simulink library "fuzblock"  (Simulink 6.0)
settings: Solver=ode45  SolverMode=SingleTasking  StartTime=0.0  StopTime=10.0  RelTol=1e-3
values from neighbouring files (symbols this model uses):
  fis = setfis(fis,'ruleList',newRuleList)    [addrule.m]    (also in anfsedit.m = get(gcbf,'UserData'); cmfdlg.m = addmf(fis,varType,varIndex,mfName,mfType,mfParams); cmthdlg.m = setfield(fis,methodType,methodName); fisgui.m = oldfis{1})
libraries: fuzblock x6
settings Model: CovMetricSettings=d  Creator=sanjai  LastModifiedBy=pascal  ProdHWDeviceType=Specified
settings DataIOCC: SignalLoggingName=logsOut
settings OptimizationCC: BooleanDataType=off
settings DebuggingCC: CheckExecutionContextPreStartOutputMsg=on  CheckExecutionContextRuntimeOutputMsg=on  SolverPrmCheckMsg=none
settings HardwareCC: ProdHWDeviceType=Specified
settings GRTTargetCC: UtilityFuncGeneration=Automatic  LifeSpan=inf
settings SFSimCC: SFSimApplyToAllLibs=on  SFSimBuildMode=Incremental

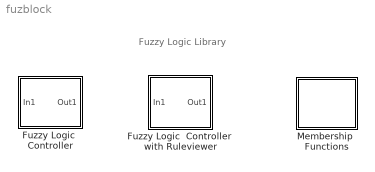
== system fuzblock ==
  note: Fuzzy Logic Library
  Fuzzy Logic  Controller : Subsystem  EnableExecutionContextPropagation=on  mask(FIS){fis=}
      mask prompts: fis "FIS File or Structure:"
      mask help: FIS
      mask init:
      | fis = fuzblockmask(gcb,fis);
      mask Help: web(['file:///' docroot '/toolbox/fuzzy/fuzzylogiccontroller.html']);
      mask Display: plot(0, -0.3, 6, -0.3, 0, 1.2, 6, 1.2, [0 6], [0 0], [1 2 3],[0 1 0],[2 3 4],[0 1 0],[3 4 5],[0 1 0])
  Fuzzy Logic  Controller  with Ruleviewer : Subsystem  EnableExecutionContextPropagation=on  mask(FIS){fismatrix=fis, Ts=2}
      mask prompts: fismatrix "FIS matrix"; Ts "Refresh rate (sec)"
      mask help: FIS with a ruleviewer for fuzzy logic rules.
      mask Help: web(['file:///' docroot '/toolbox/fuzzy/fuzzylogiccontrollerwithr.html']);
      mask Display: plot(0, -0.3, 6, -0.3, 0, 1.2, 6, 1.2, [0 6], [0 0], [1 2 3],[0 1 0],[2 3 4],[0 1 0],[3 4 5],[0 1 0])
  Membership  Functions : Subsystem  EnableExecutionContextPropagation=on
      mask Type: MF Library
      mask Display: disp('MF')

== system fuzblock/Fuzzy Logic  Controller ==
  In1 : Inport  LatchInput=off
  FIS S-function : S-Function  FunctionName=sffis  Parameters=fis  SFunctionModules=sfsup
  Out1 : Outport
  wires:
  FIS S-function/1 -> Out1/1
  In1/1 -> FIS S-function/1

== system fuzblock/Fuzzy Logic  Controller  with Ruleviewer ==
  In1 : Inport  LatchInput=off
  Animation1 : S-Function  FunctionName=animrule  Parameters=fismatrix
  Fuzzy Logic Controller : fuzblock/Fuzzy Logic  Controller  fis=fismatrix
  Zero-Order Hold : ZeroOrderHold  SampleTime=Ts
  Out1 : Outport  InitialOutput=0
  wires:
  Zero-Order Hold/1 -> Animation1/1
  Fuzzy Logic Controller/1 -> Out1/1
  In1/1 -> Fuzzy Logic Controller/1, Zero-Order Hold/1

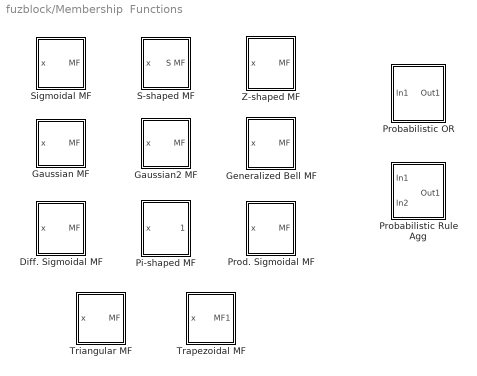
== system fuzblock/Membership  Functions ==
  Diff. Sigmoidal MF : Subsystem  EnableExecutionContextPropagation=on  mask(dsigmf){a1=3, c1=-5, a2=1, c2=5}
      mask prompts: a1 "Left curve a1:"; c1 "Left curve c1:"; a2 "Right curve a2:"; c2 "Right curve c2:"
      mask help:
      | "Difference of two sigmoids" membership function. The two sigmoid curves are given by
      |
      |         fk ( x ) = 1 / ( 1 + exp( -ak ( x - ck) ) )      k=1,2
      |
      | The parameters a1 and a2 control the slopes of the left and right curves. The parameters c1 and c2 control the points of inflection for the left and right curves. The parameters a1 and a2 should be positive.
      mask init:
      | x=-10:0.5:10;
      | params=[3 -5 1 5];
      | y=dsigmf(x,params);
      mask Help: web(['file:///' docroot '/toolbox/fuzzy/membershipfunctionslibrar.html']);
      mask Display: plot(x,y);
  Gaussian MF : Subsystem  EnableExecutionContextPropagation=on  mask(gaussmf){sigma=1, mu=0}
      mask prompts: sigma "Variance sigma:"; mu "Mean c:"
      mask help:
      | Symmetric Gaussian membership function given by
      |
      |         f ( x ) = exp ^ ( ( - 0.5 ( x - c) ^ 2 ) / sigma ^ 2 )
      |
      | where c is the mean and sigma is the variance.
      mask init:
      | x=-10:0.5:10;
      | params=[7 0];
      | y=gaussmf(x,params);
      mask Help: web(['file:///' docroot '/toolbox/fuzzy/membershipfunctionslibrar.html']);
      mask Display: plot(x,y);
  Gaussian2 MF : Subsystem  EnableExecutionContextPropagation=on  mask(gauss2mf){sigma1=3, mu1=-1, sigma2=1, mu2=5}
      mask prompts: sigma1 "Variance for left curve sigma1:"; mu1 "Mean for left curve c1:"; sigma2 "Variance for right curve sigma2:"; mu2 "Mean for right curve c2:"
      mask help:
      | "Combination of two Gaussians" membership function. The two Gaussian functions are given by
      |
      |         fk ( x ) = exp ^ ( ( - 0.5 ( x - ck) ^ 2 ) / sigmak ^ 2 )    k=1,2
      |
      | The parameters c1 and sigma1 are the mean and variance defining the leftmost curve. The parameters c2 and sigma2 are the mean and variance defining the rightmost curve.
      mask init:
      | x=-10:0.5:10;
      | params=[3 -1 1 5];
      | y=gauss2mf(x,params);
      mask Help: web(['file:///' docroot '/toolbox/fuzzy/membershipfunctionslibrar.html']);
      mask Display: plot(x,y);
  Generalized Bell MF : Subsystem  EnableExecutionContextPropagation=on  mask(gbellmf){a=5, b=4, c=0}
      mask help:
      | Generalized bell membership function given by
      |
      |         f ( x ) = 1 / ( 1 + | ( x - c) / a | ^ 2b )
      |
      | The parameters a and b vary the width of the curve and the parameter c locates the center of the curve. The parameter b should be positive.
      mask init:
      | x=-10:0.5:10;
      | params=[5 4 0];
      | y=gbellmf(x,params);
      mask Help: web(['file:///' docroot '/toolbox/fuzzy/membershipfunctionslibrar.html']);
      mask Display: plot(x,y);
  Pi-shaped MF : Subsystem  EnableExecutionContextPropagation=on  mask(pimf){a=-9, b=-7, c=2, d=8}
      mask prompts: a "Left base point a:"; b "Left top point b:"; c "Right top point c:"; d "Right base point d:"
      mask help:
      | Pi-shaped membership function.
      |
      | The parameters a and d  set the left and right base point or "feet" of the curve.  The parameters b and c set the left and right top point or "shoulders" of the curve.
      mask init:
      | x=-10:0.5:10;
      | params=[-9 -7 2 8];
      | y=pimf(x,params);
      mask Help: web(['file:///' docroot '/toolbox/fuzzy/membershipfunctionslibrar.html']);
      mask Display: plot(x,y);
  Probabilistic OR : Subsystem  EnableExecutionContextPropagation=on
      mask Type: probor OR method
      mask Description:
      | Probabilistic OR function.
      | 
      |         y = 1 - prod( 1 - x )
      | 
      | This block outputs the probabilistic OR value for the vector signal input.
      mask Help: web(['file:///' docroot '/toolbox/fuzzy/membershipfunctionslibrar.html']);
      mask Display: disp('Probor')
  Probabilistic Rule Agg : Subsystem  EnableExecutionContextPropagation=on
      mask Type: probor rule agg method
      mask Description:
      | Probabilistic OR, rule aggregation method.
      | 
      |         y = 1 - prod( 1 - [ a ; b ] )
      | 
      | This block outputs the element-wise(.*) probabilistic OR value of the two inputs. The two inputs a and b, are row vectors.
      mask Help: web(['file:///' docroot '/toolbox/fuzzy/membershipfunctionslibrar.html']);
      mask Display: disp('Probor')
  Prod. Sigmoidal MF : Subsystem  EnableExecutionContextPropagation=on  mask(psigmf){a1=2, c1=-5, a2=-5, c2=5}
      mask prompts: a1 "Left curve a1:"; c1 "Left curve c1:"; a2 "Right curve a2:"; c2 "Right curve c2:"
      mask help:
      | "Product of two sigmoids" membership function. The two sigmoid curves are given by
      |
      |         fk ( x ) = 1 / ( 1 + exp( -ak ( x - ck) ) )      k=1,2
      |
      | The parameters a1 and a2 control the slopes of the left and right curves. The parameters c1 and c2 control the points of inflection for the left and right curves. Parameters a1 and a2 should be positive and negative respectively.
      mask init:
      | x=-10:0.5:10;
      | params=[2 -5 -5 5];
      | y=psigmf(x,params);
      mask Help: web(['file:///' docroot '/toolbox/fuzzy/membershipfunctionslibrar.html']);
      mask Display: plot(x,y);
  S-shaped MF : Subsystem  EnableExecutionContextPropagation=on  mask(smf){a=-3, b=3}
      mask prompts: a "Left point a:"; b "Right point b:"
      mask help:
      | S-shaped membership function.
      |
      | Going from left to right the function increases from 0 to 1. The parameters a and b locate the left and right extremes of the sloped portion of the curve.
      mask init:
      | x=-10:0.5:10;
      | params=[-3 3];
      | y=smf(x,params);
      mask Help: web(['file:///' docroot '/toolbox/fuzzy/membershipfunctionslibrar.html']);
      mask Display: plot(x,y);
  Sigmoidal MF : Subsystem  EnableExecutionContextPropagation=on  mask(sigmf){a=1, c=0}
      mask help:
      | Sigmoidal membership function given by
      |
      |         f ( x ) = 1 / ( 1 + exp( -a ( x - c) ) )
      |
      | When the sign of a is positive the curve increases from left to right. Conversely, when the sign of a is negative the curve decreases from left to right. The parameter c sets the point of inflection of the curve.
      mask init:
      | x=-10:0.5:10;
      | params=[1 0];
      | y=sigmf(x,params);
      mask Help: web(['file:///' docroot '/toolbox/fuzzy/membershipfunctionslibrar.html']);
      mask Display: plot(x,y);
  Trapezoidal MF : Subsystem  EnableExecutionContextPropagation=on  mask(trapmf){a=-8, b=-4, c=2, d=9}
      mask prompts: a "Left base point a:"; b "Left top point b:"; c "Right top point c:"; d "Right base point d:"
      mask help:
      | Trapezoidal membership function.
      |
      | The parameters a and d set the left and right "feet", or base points, of the trapezoid. The parameters b and c set the "shoulders", or top of the trapezoid.
      mask init:
      | x=-10:0.5:10;
      | params=[-8 -4 2 9];
      | y=trapmf(x,params);
      mask Help: web(['file:///' docroot '/toolbox/fuzzy/membershipfunctionslibrar.html']);
      mask Display: plot(x,y);
  Triangular MF : Subsystem  EnableExecutionContextPropagation=on  mask(trimf){a=-8, b=3, c=6}
      mask prompts: a "Left base point a:"; b "Peak location b:"; c "Right base point c:"
      mask help:
      | Triangular membership function.
      |
      | The parameters a and c set the left and right "feet", or base points, of the triangle. The parameter b sets the location of the triangle peak.
      mask init:
      | x=-10:0.5:10;
      | params=[-8 3 6];
      | y=trimf(x,params);
      mask Help: web(['file:///' docroot '/toolbox/fuzzy/membershipfunctionslibrar.html']);
      mask Display: plot(x,y);
  Z-shaped MF : Subsystem  EnableExecutionContextPropagation=on  mask(zmf){a=-3, b=3}
      mask prompts: a "Left point a:"; b "Right point b:"
      mask help:
      | Z-shaped membership function.
      |
      | Going from left to right the function decreases from 1 to 0. The parameters a  and b locate the left and right extremes of the sloped portion of the curve.
      mask init:
      | x=-10:0.5:10;
      | params=[-3 3];
      | y=zmf(x,params);
      mask Help: web(['file:///' docroot '/toolbox/fuzzy/membershipfunctionslibrar.html']);
      mask Display: plot(x,y);

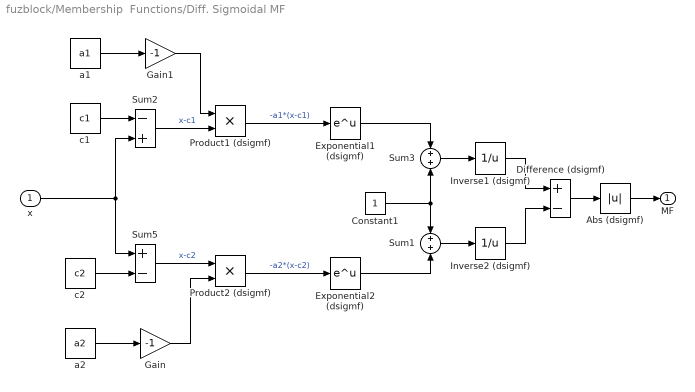
== system fuzblock/Membership  Functions/Diff. Sigmoidal MF ==
  x : Inport  LatchInput=off
  Abs (dsigmf) : Abs  ZeroCross=off  SaturateOnIntegerOverflow=on
  Constant1 : Constant
  Difference (dsigmf) : Sum  Inputs=+-  SaturateOnIntegerOverflow=on  InputSameDT=on
  Exponential1 (dsigmf) : Math  SaturateOnIntegerOverflow=on
  Exponential2 (dsigmf) : Math  SaturateOnIntegerOverflow=on
  Gain : Gain  Gain=-1  SaturateOnIntegerOverflow=on
  Gain1 : Gain  Gain=-1  SaturateOnIntegerOverflow=on
  Inverse1 (dsigmf) : Math  Operator=reciprocal  SaturateOnIntegerOverflow=on
  Inverse2 (dsigmf) : Math  Operator=reciprocal  SaturateOnIntegerOverflow=on
  Product1 (dsigmf) : Product  Inputs=**  SaturateOnIntegerOverflow=on  InputSameDT=on
  Product2 (dsigmf) : Product  Inputs=**  SaturateOnIntegerOverflow=on  InputSameDT=on
  Sum1 : Sum  SaturateOnIntegerOverflow=on  InputSameDT=on
  Sum2 : Sum  Inputs=-+  SaturateOnIntegerOverflow=on  InputSameDT=on
  Sum3 : Sum  SaturateOnIntegerOverflow=on  InputSameDT=on
  Sum5 : Sum  Inputs=+-  SaturateOnIntegerOverflow=on  InputSameDT=on
  a1 : Constant  Value=a1
  a2 : Constant  Value=a2
  c1 : Constant  Value=c1
  c2 : Constant  Value=c2
  MF : Outport
  wires:
  Abs (dsigmf)/1 -> MF/1
  Difference (dsigmf)/1 -> Abs (dsigmf)/1
  Inverse2 (dsigmf)/1 -> Difference (dsigmf)/2
  Inverse1 (dsigmf)/1 -> Difference (dsigmf)/1
  Gain1/1 -> Product1 (dsigmf)/1
  a1/1 -> Gain1/1
  Constant1/1 -> Sum1/1, Sum3/2
  Exponential2 (dsigmf)/1 -> Sum1/2
  Product1 (dsigmf)/1 -> Exponential1 (dsigmf)/1  "-a1*(x-c1)"
  Sum2/1 -> Product1 (dsigmf)/2  "x-c1"
  c1/1 -> Sum2/1
  Exponential1 (dsigmf)/1 -> Sum3/1
  Sum3/1 -> Inverse1 (dsigmf)/1
  Gain/1 -> Product2 (dsigmf)/2
  a2/1 -> Gain/1
  Product2 (dsigmf)/1 -> Exponential2 (dsigmf)/1  "-a2*(x-c2)"
  Sum5/1 -> Product2 (dsigmf)/1  "x-c2"
  c2/1 -> Sum5/2
  Sum1/1 -> Inverse2 (dsigmf)/1
  x/1 -> Sum5/1, Sum2/2

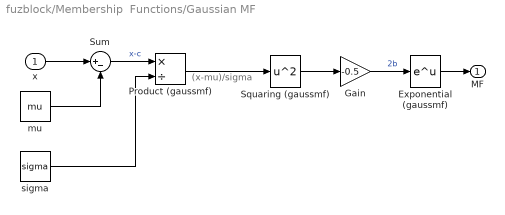
== system fuzblock/Membership  Functions/Gaussian MF ==
  note: (x-mu)/sigma
  x : Inport  LatchInput=off
  Exponential (gaussmf) : Math  SaturateOnIntegerOverflow=on
  Gain : Gain  Gain=-0.5  SaturateOnIntegerOverflow=on
  Product (gaussmf) : Product  Inputs=*/  SaturateOnIntegerOverflow=on  InputSameDT=on
  Squaring (gaussmf) : Math  Operator=square  SaturateOnIntegerOverflow=on
  Sum : Sum  Inputs=|+-  SaturateOnIntegerOverflow=on  InputSameDT=on
  mu : Constant  Value=mu
  sigma : Constant  Value=sigma
  MF : Outport
  wires:
  x/1 -> Sum/1
  mu/1 -> Sum/2
  Sum/1 -> Product (gaussmf)/1  "x-c"
  sigma/1 -> Product (gaussmf)/2
  Exponential (gaussmf)/1 -> MF/1
  Squaring (gaussmf)/1 -> Gain/1
  Gain/1 -> Exponential (gaussmf)/1  "2b"
  Product (gaussmf)/1 -> Squaring (gaussmf)/1

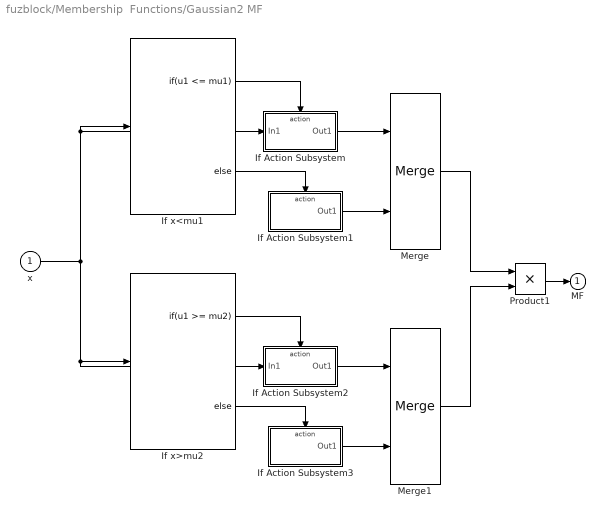
== system fuzblock/Membership  Functions/Gaussian2 MF ==
  x : Inport  LatchInput=off
  If Action Subsystem : Subsystem  TreatAsAtomicUnit=on  EnableExecutionContextPropagation=on
  If Action Subsystem1 : Subsystem  TreatAsAtomicUnit=on  EnableExecutionContextPropagation=on
  If Action Subsystem2 : Subsystem  TreatAsAtomicUnit=on  EnableExecutionContextPropagation=on
  If Action Subsystem3 : Subsystem  TreatAsAtomicUnit=on  EnableExecutionContextPropagation=on
  If x<mu1 : If  IfExpression=u1 <= mu1  ZeroCross=off
  If x>mu2 : If  IfExpression=u1 >= mu2  ZeroCross=off
  Merge : Merge
  Merge1 : Merge
  Product1 : Product  SaturateOnIntegerOverflow=on  InputSameDT=on
  MF : Outport
  wires:
  If x<mu1/1 -> If Action Subsystem/Action
  Merge/1 -> Product1/1
  If Action Subsystem/1(Out1) -> Merge/1
  If x<mu1/2 -> If Action Subsystem1/Action
  If Action Subsystem1/1(Out1) -> Merge/2
  Product1/1 -> MF/1
  If x>mu2/1 -> If Action Subsystem2/Action
  If Action Subsystem2/1(Out1) -> Merge1/1
  If x>mu2/2 -> If Action Subsystem3/Action
  If Action Subsystem3/1(Out1) -> Merge1/2
  Merge1/1 -> Product1/2
  x/1 -> If x<mu1/1, If Action Subsystem/1(In1), If x>mu2/1, If Action Subsystem2/1(In1)

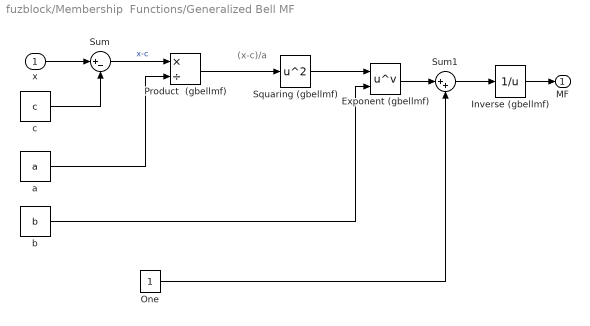
== system fuzblock/Membership  Functions/Generalized Bell MF ==
  note: (x-c)/a
  x : Inport  LatchInput=off
  Exponent (gbellmf) : Math  Operator=pow  SaturateOnIntegerOverflow=on
  Inverse (gbellmf) : Math  Operator=reciprocal  SaturateOnIntegerOverflow=on
  One : Constant
  Product  (gbellmf) : Product  Inputs=*/  SaturateOnIntegerOverflow=on  InputSameDT=on
  Squaring (gbellmf) : Math  Operator=square  SaturateOnIntegerOverflow=on
  Sum : Sum  Inputs=|+-  SaturateOnIntegerOverflow=on  InputSameDT=on
  Sum1 : Sum  Inputs=|++  SaturateOnIntegerOverflow=on  InputSameDT=on
  a : Constant  Value=a
  b : Constant  Value=b
  c : Constant  Value=c
  MF : Outport
  wires:
  b/1 -> Exponent (gbellmf)/2
  Squaring (gbellmf)/1 -> Exponent (gbellmf)/1
  Product  (gbellmf)/1 -> Squaring (gbellmf)/1
  a/1 -> Product  (gbellmf)/2
  Sum/1 -> Product  (gbellmf)/1  "x-c"
  c/1 -> Sum/2
  x/1 -> Sum/1
  Exponent (gbellmf)/1 -> Sum1/1
  One/1 -> Sum1/2
  Sum1/1 -> Inverse (gbellmf)/1
  Inverse (gbellmf)/1 -> MF/1

== system fuzblock/Membership  Functions/Pi-shaped MF ==
  x : Inport  LatchInput=off
  Constant4 : Constant
  Product : Product  SaturateOnIntegerOverflow=on  InputSameDT=on
  Sum : Sum  Inputs=-+  SaturateOnIntegerOverflow=on  InputSameDT=on
  Z-shaped MF : fuzblock/Membership  Functions/Z-shaped MF  a=a  b=b
  Z-shaped MF1 : fuzblock/Membership  Functions/Z-shaped MF  a=c  b=d
  Pi MF : Outport
  wires:
  Product/1 -> Pi MF/1
  Z-shaped MF1/1 -> Product/2  "Z MF"
  x/1 -> Z-shaped MF/1, Z-shaped MF1/1
  Z-shaped MF/1 -> Sum/1
  Constant4/1 -> Sum/2
  Sum/1 -> Product/1  "S MF"

== system fuzblock/Membership  Functions/Probabilistic OR ==
  note: probor ( X) = 1-prod(1-X)
  note: X
  In1 : Inport  LatchInput=off
  Constant4 : Constant
  Product : Product  Inputs=1  SaturateOnIntegerOverflow=on  InputSameDT=on
  Sum : Sum  Inputs=-+  SaturateOnIntegerOverflow=on  InputSameDT=on
  Sum1 : Sum  Inputs=-+  SaturateOnIntegerOverflow=on  InputSameDT=on
  Out1 : Outport
  wires:
  Sum1/1 -> Out1/1
  In1/1 -> Sum/1
  Constant4/1 -> Sum1/2, Sum/2
  Sum/1 -> Product/1
  Product/1 -> Sum1/1

== system fuzblock/Membership  Functions/Probabilistic Rule Agg ==
  note: probor ( [a; b] ) = 1-prod(1-[a;b])
  note: a
  note: b
  In1 : Inport  LatchInput=off
  In2 : Inport  Port=2  LatchInput=off
  Product : Product  SaturateOnIntegerOverflow=on  InputSameDT=on
  Sum : Sum  SaturateOnIntegerOverflow=on  InputSameDT=on
  Sum1 : Sum  Inputs=+-  SaturateOnIntegerOverflow=on  InputSameDT=on
  Out1 : Outport
  wires:
  Sum1/1 -> Out1/1
  In1/1 -> Sum/1, Product/1
  In2/1 -> Sum/2, Product/2
  Sum/1 -> Sum1/1
  Product/1 -> Sum1/2

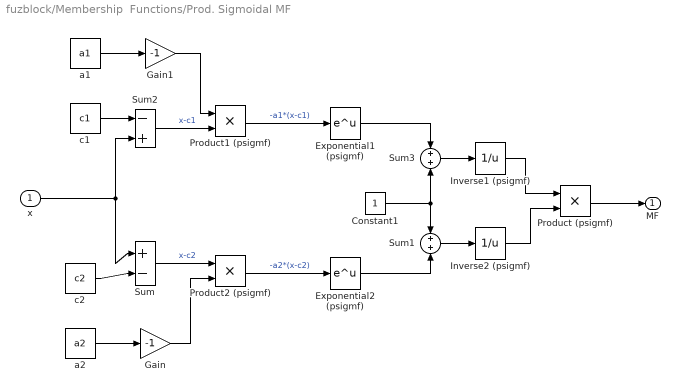
== system fuzblock/Membership  Functions/Prod. Sigmoidal MF ==
  x : Inport  LatchInput=off
  Constant1 : Constant
  Exponential1 (psigmf) : Math  SaturateOnIntegerOverflow=on
  Exponential2 (psigmf) : Math  SaturateOnIntegerOverflow=on
  Gain : Gain  Gain=-1  SaturateOnIntegerOverflow=on
  Gain1 : Gain  Gain=-1  SaturateOnIntegerOverflow=on
  Inverse1 (psigmf) : Math  Operator=reciprocal  SaturateOnIntegerOverflow=on
  Inverse2 (psigmf) : Math  Operator=reciprocal  SaturateOnIntegerOverflow=on
  Product (psigmf) : Product  Inputs=**  SaturateOnIntegerOverflow=on  InputSameDT=on
  Product1 (psigmf) : Product  Inputs=**  SaturateOnIntegerOverflow=on  InputSameDT=on
  Product2 (psigmf) : Product  Inputs=**  SaturateOnIntegerOverflow=on  InputSameDT=on
  Sum : Sum  Inputs=|+-  SaturateOnIntegerOverflow=on  InputSameDT=on
  Sum1 : Sum  SaturateOnIntegerOverflow=on  InputSameDT=on
  Sum2 : Sum  Inputs=-+  SaturateOnIntegerOverflow=on  InputSameDT=on
  Sum3 : Sum  SaturateOnIntegerOverflow=on  InputSameDT=on
  a1 : Constant  Value=a1
  a2 : Constant  Value=a2
  c1 : Constant  Value=c1
  c2 : Constant  Value=c2
  MF : Outport
  wires:
  Gain1/1 -> Product1 (psigmf)/1
  a1/1 -> Gain1/1
  Constant1/1 -> Sum1/1, Sum3/2
  Exponential2 (psigmf)/1 -> Sum1/2
  Inverse1 (psigmf)/1 -> Product (psigmf)/1
  Product1 (psigmf)/1 -> Exponential1 (psigmf)/1  "-a1*(x-c1)"
  Sum2/1 -> Product1 (psigmf)/2  "x-c1"
  c1/1 -> Sum2/1
  Exponential1 (psigmf)/1 -> Sum3/1
  Sum3/1 -> Inverse1 (psigmf)/1
  Inverse2 (psigmf)/1 -> Product (psigmf)/2
  Gain/1 -> Product2 (psigmf)/2
  a2/1 -> Gain/1
  Product2 (psigmf)/1 -> Exponential2 (psigmf)/1  "-a2*(x-c2)"
  Sum/1 -> Product2 (psigmf)/1  "x-c2"
  c2/1 -> Sum/2
  Sum1/1 -> Inverse2 (psigmf)/1
  Product (psigmf)/1 -> MF/1
  x/1 -> Sum/1, Sum2/2

== system fuzblock/Membership  Functions/S-shaped MF ==
  x : Inport  LatchInput=off
  Constant4 : Constant
  Sum : Sum  Inputs=-+  SaturateOnIntegerOverflow=on  InputSameDT=on
  Z-shaped MF : fuzblock/Membership  Functions/Z-shaped MF  a=a  b=b
  S MF : Outport
  wires:
  x/1 -> Z-shaped MF/1
  Sum/1 -> S MF/1
  Constant4/1 -> Sum/2
  Z-shaped MF/1 -> Sum/1

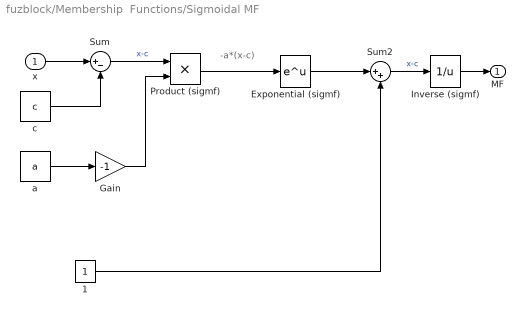
== system fuzblock/Membership  Functions/Sigmoidal MF ==
  note: -a*(x-c)
  x : Inport  LatchInput=off
  1 : Constant
  Exponential (sigmf) : Math  SaturateOnIntegerOverflow=on
  Gain : Gain  Gain=-1  SaturateOnIntegerOverflow=on
  Inverse (sigmf) : Math  Operator=reciprocal  SaturateOnIntegerOverflow=on
  Product (sigmf) : Product  Inputs=**  SaturateOnIntegerOverflow=on  InputSameDT=on
  Sum : Sum  Inputs=|+-  SaturateOnIntegerOverflow=on  InputSameDT=on
  Sum2 : Sum  Inputs=|++  SaturateOnIntegerOverflow=on  InputSameDT=on
  a : Constant  Value=a
  c : Constant  Value=c
  MF : Outport
  wires:
  Gain/1 -> Product (sigmf)/2
  a/1 -> Gain/1
  Product (sigmf)/1 -> Exponential (sigmf)/1
  Sum/1 -> Product (sigmf)/1  "x-c"
  c/1 -> Sum/2
  x/1 -> Sum/1
  1/1 -> Sum2/2
  Sum2/1 -> Inverse (sigmf)/1  "x-c"
  Inverse (sigmf)/1 -> MF/1
  Exponential (sigmf)/1 -> Sum2/1

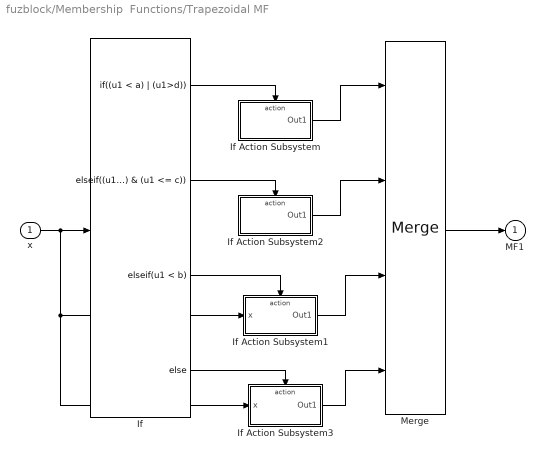
== system fuzblock/Membership  Functions/Trapezoidal MF ==
  x : Inport  LatchInput=off
  If : If  IfExpression=(u1 < a) | (u1>d)  ElseIfExpressions=(u1 >= b) & (u1 <= c), u1 < b  ZeroCross=off
  If Action Subsystem : Subsystem  TreatAsAtomicUnit=on  EnableExecutionContextPropagation=on
  If Action Subsystem1 : Subsystem  TreatAsAtomicUnit=on  EnableExecutionContextPropagation=on
  If Action Subsystem2 : Subsystem  TreatAsAtomicUnit=on  EnableExecutionContextPropagation=on
  If Action Subsystem3 : Subsystem  TreatAsAtomicUnit=on  EnableExecutionContextPropagation=on
  Merge : Merge  Inputs=4
  MF1 : Outport
  wires:
  If/1 -> If Action Subsystem/Action
  Merge/1 -> MF1/1
  If Action Subsystem/1(Out1) -> Merge/1
  If/4 -> If Action Subsystem3/Action
  If/3 -> If Action Subsystem1/Action
  x/1 -> If/1, If Action Subsystem1/1(x), If Action Subsystem3/1(x)
  If/2 -> If Action Subsystem2/Action
  If Action Subsystem2/1(Out1) -> Merge/2
  If Action Subsystem1/1(Out1) -> Merge/3
  If Action Subsystem3/1(Out1) -> Merge/4

== system fuzblock/Membership  Functions/Triangular MF ==
  x : Inport  LatchInput=off
  If : If  IfExpression=(u1<a) | (u1>c)  ElseIfExpressions=u1==b, u1 < b  ZeroCross=off
  If Action Subsystem : Subsystem  TreatAsAtomicUnit=on  EnableExecutionContextPropagation=on
  If Action Subsystem1 : Subsystem  TreatAsAtomicUnit=on  EnableExecutionContextPropagation=on
  If Action Subsystem2 : Subsystem  TreatAsAtomicUnit=on  EnableExecutionContextPropagation=on
  If Action Subsystem3 : Subsystem  TreatAsAtomicUnit=on  EnableExecutionContextPropagation=on
  Merge : Merge  Inputs=4
  MF : Outport
  wires:
  x/1 -> If/1, If Action Subsystem2/1(x), If Action Subsystem3/1(x)
  If/1 -> If Action Subsystem/Action
  Merge/1 -> MF/1
  If Action Subsystem/1(Out1) -> Merge/1
  If/2 -> If Action Subsystem1/Action
  If Action Subsystem1/1(Out1) -> Merge/2
  If/4 -> If Action Subsystem2/Action
  If Action Subsystem2/1(Out1) -> Merge/4
  If/3 -> If Action Subsystem3/Action
  If Action Subsystem3/1(Out1) -> Merge/3

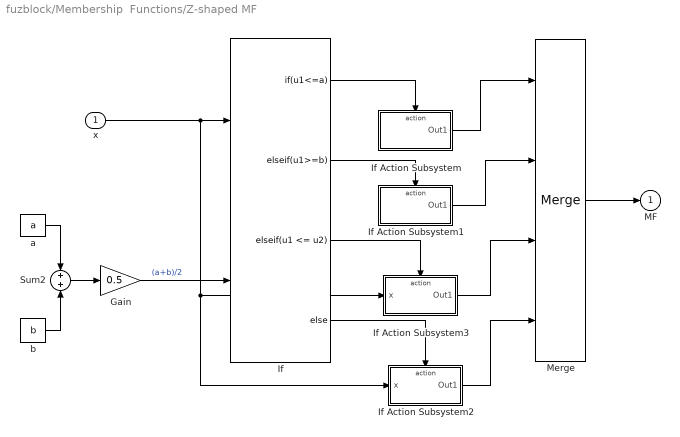
== system fuzblock/Membership  Functions/Z-shaped MF ==
  x : Inport  LatchInput=off
  Gain : Gain  Gain=0.5  SaturateOnIntegerOverflow=on
  If : If  NumInputs=2  IfExpression=u1<=a  ElseIfExpressions=u1>=b, u1 <= u2  ZeroCross=off
  If Action Subsystem : Subsystem  TreatAsAtomicUnit=on  EnableExecutionContextPropagation=on
  If Action Subsystem1 : Subsystem  TreatAsAtomicUnit=on  EnableExecutionContextPropagation=on
  If Action Subsystem2 : Subsystem  TreatAsAtomicUnit=on  EnableExecutionContextPropagation=on
  If Action Subsystem3 : Subsystem  TreatAsAtomicUnit=on  EnableExecutionContextPropagation=on
  Merge : Merge  Inputs=4
  Sum2 : Sum  SaturateOnIntegerOverflow=on  InputSameDT=on
  a : Constant  Value=a
  b : Constant  Value=b
  MF : Outport
  wires:
  If/1 -> If Action Subsystem/Action
  Merge/1 -> MF/1
  If Action Subsystem/1(Out1) -> Merge/1
  If/2 -> If Action Subsystem1/Action
  If Action Subsystem1/1(Out1) -> Merge/2
  If/4 -> If Action Subsystem2/Action
  If Action Subsystem2/1(Out1) -> Merge/4
  If/3 -> If Action Subsystem3/Action
  If Action Subsystem3/1(Out1) -> Merge/3
  x/1 -> If/1, If Action Subsystem3/1(x), If Action Subsystem2/1(x)
  a/1 -> Sum2/1
  b/1 -> Sum2/2
  Sum2/1 -> Gain/1
  Gain/1 -> If/2  "(a+b)/2"

== system fuzblock/Membership  Functions/Gaussian2 MF/If Action Subsystem ==
  In1 : Inport  LatchInput=off
  Action Port : ActionPort
  Gaussian MF : fuzblock/Membership  Functions/Gaussian MF  sigma=sigma1  mu=mu1
  Out1 : Outport  InitialOutput=0
  wires:
  In1/1 -> Gaussian MF/1
  Gaussian MF/1 -> Out1/1

== system fuzblock/Membership  Functions/Gaussian2 MF/If Action Subsystem1 ==
  Action Port : ActionPort
  0 : Constant
  Out1 : Outport  InitialOutput=1
  wires:
  0/1 -> Out1/1

== system fuzblock/Membership  Functions/Gaussian2 MF/If Action Subsystem2 ==
  In1 : Inport  LatchInput=off
  Action Port : ActionPort
  Gaussian MF : fuzblock/Membership  Functions/Gaussian MF  sigma=sigma2  mu=mu2
  Out1 : Outport  InitialOutput=0
  wires:
  Gaussian MF/1 -> Out1/1
  In1/1 -> Gaussian MF/1

== system fuzblock/Membership  Functions/Gaussian2 MF/If Action Subsystem3 ==
  Action Port : ActionPort
  0 : Constant
  Out1 : Outport  InitialOutput=1
  wires:
  0/1 -> Out1/1

== system fuzblock/Membership  Functions/Trapezoidal MF/If Action Subsystem ==
  Action Port : ActionPort
  0 : Constant  Value=0
  Out1 : Outport  InitialOutput=0
  wires:
  0/1 -> Out1/1

== system fuzblock/Membership  Functions/Trapezoidal MF/If Action Subsystem1 ==
  x : Inport  LatchInput=off
  Action Port : ActionPort
  Product ab (trimf) : Product  Inputs=*/  SaturateOnIntegerOverflow=on  InputSameDT=on
  Sum : Sum  Inputs=|+-  SaturateOnIntegerOverflow=on  InputSameDT=on
  Sum1 : Sum  Inputs=-+  SaturateOnIntegerOverflow=on  InputSameDT=on
  a : Constant  Value=a
  b : Constant  Value=b
  Out1 : Outport
  wires:
  Product ab (trimf)/1 -> Out1/1  "(x-a)/(b-a)"
  a/1 -> Sum/2, Sum1/1
  b/1 -> Sum1/2
  x/1 -> Sum/1
  Sum/1 -> Product ab (trimf)/1  "x-a"
  Sum1/1 -> Product ab (trimf)/2  "b-a"

== system fuzblock/Membership  Functions/Trapezoidal MF/If Action Subsystem2 ==
  Action Port : ActionPort  ActionType=elseif
  0 : Constant
  Out1 : Outport  InitialOutput=0
  wires:
  0/1 -> Out1/1

== system fuzblock/Membership  Functions/Trapezoidal MF/If Action Subsystem3 ==
  x : Inport  LatchInput=off
  Action Port : ActionPort  ActionType=else
  Product cd (trimf) : Product  Inputs=/*  SaturateOnIntegerOverflow=on  InputSameDT=on
  Sum2 : Sum  Inputs=-+  SaturateOnIntegerOverflow=on  InputSameDT=on
  Sum3 : Sum  Inputs=+-  SaturateOnIntegerOverflow=on  InputSameDT=on
  c : Constant  Value=c
  d : Constant  Value=d
  Out1 : Outport
  wires:
  Product cd (trimf)/1 -> Out1/1  "(d-x)/(d-c)"
  Sum2/1 -> Product cd (trimf)/1  "d-c"
  Sum3/1 -> Product cd (trimf)/2  "d-x"
  d/1 -> Sum2/2, Sum3/1
  x/1 -> Sum3/2
  c/1 -> Sum2/1

== system fuzblock/Membership  Functions/Triangular MF/If Action Subsystem ==
  Action Port : ActionPort  ActionType=then
  0 : Constant  Value=0
  Out1 : Outport  InitialOutput=0
  wires:
  0/1 -> Out1/1

== system fuzblock/Membership  Functions/Triangular MF/If Action Subsystem1 ==
  Action Port : ActionPort  ActionType=elseif
  0 : Constant
  Out1 : Outport  InitialOutput=1
  wires:
  0/1 -> Out1/1

== system fuzblock/Membership  Functions/Triangular MF/If Action Subsystem2 ==
  x : Inport  LatchInput=off
  Action Port : ActionPort  ActionType=else
  Product cd (trimf) : Product  Inputs=/*  SaturateOnIntegerOverflow=on  InputSameDT=on
  Sum2 : Sum  Inputs=-+  SaturateOnIntegerOverflow=on  InputSameDT=on
  Sum3 : Sum  Inputs=+-  SaturateOnIntegerOverflow=on  InputSameDT=on
  b : Constant  Value=b
  c : Constant  Value=c
  Out1 : Outport
  wires:
  Product cd (trimf)/1 -> Out1/1  "(c-x)/(c-b)"
  Sum2/1 -> Product cd (trimf)/1  "c-b"
  Sum3/1 -> Product cd (trimf)/2  "c-x"
  c/1 -> Sum2/2, Sum3/1
  x/1 -> Sum3/2
  b/1 -> Sum2/1

== system fuzblock/Membership  Functions/Triangular MF/If Action Subsystem3 ==
  x : Inport  LatchInput=off
  Action Port : ActionPort  ActionType=elseif
  Product ab (trimf) : Product  Inputs=*/  SaturateOnIntegerOverflow=on  InputSameDT=on
  Sum : Sum  Inputs=|+-  SaturateOnIntegerOverflow=on  InputSameDT=on
  Sum1 : Sum  Inputs=-+  SaturateOnIntegerOverflow=on  InputSameDT=on
  a : Constant  Value=a
  b : Constant  Value=b
  Out1 : Outport
  wires:
  Sum1/1 -> Product ab (trimf)/2  "b-a"
  Sum/1 -> Product ab (trimf)/1  "x-a"
  x/1 -> Sum/1
  b/1 -> Sum1/2
  a/1 -> Sum/2, Sum1/1
  Product ab (trimf)/1 -> Out1/1  "(x-a)/(b-a)"

== system fuzblock/Membership  Functions/Z-shaped MF/If Action Subsystem ==
  Action Port : ActionPort
  0 : Constant
  Out1 : Outport  InitialOutput=0
  wires:
  0/1 -> Out1/1

== system fuzblock/Membership  Functions/Z-shaped MF/If Action Subsystem1 ==
  Action Port : ActionPort
  0 : Constant  Value=0
  Out1 : Outport  InitialOutput=1
  wires:
  0/1 -> Out1/1

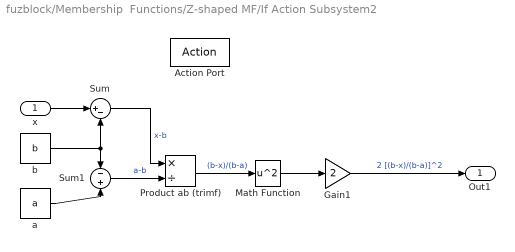
== system fuzblock/Membership  Functions/Z-shaped MF/If Action Subsystem2 ==
  x : Inport  LatchInput=off
  Action Port : ActionPort
  Gain1 : Gain  Gain=2  SaturateOnIntegerOverflow=on
  Math Function : Math  Operator=square  SaturateOnIntegerOverflow=on
  Product ab (trimf) : Product  Inputs=*/  SaturateOnIntegerOverflow=on  InputSameDT=on
  Sum : Sum  Inputs=|+-  SaturateOnIntegerOverflow=on  InputSameDT=on
  Sum1 : Sum  Inputs=-+  SaturateOnIntegerOverflow=on  InputSameDT=on
  a : Constant  Value=a
  b : Constant  Value=b
  Out1 : Outport
  wires:
  Product ab (trimf)/1 -> Math Function/1  "(b-x)/(b-a)"
  b/1 -> Sum/2, Sum1/1
  a/1 -> Sum1/2
  x/1 -> Sum/1
  Sum/1 -> Product ab (trimf)/1  "x-b"
  Sum1/1 -> Product ab (trimf)/2  "a-b"
  Math Function/1 -> Gain1/1
  Gain1/1 -> Out1/1  "2 [(b-x)/(b-a)]^2"

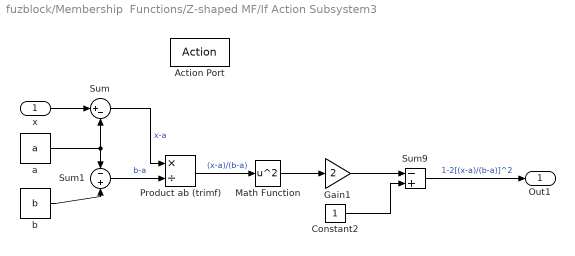
== system fuzblock/Membership  Functions/Z-shaped MF/If Action Subsystem3 ==
  x : Inport  LatchInput=off
  Action Port : ActionPort
  Constant2 : Constant
  Gain1 : Gain  Gain=2  SaturateOnIntegerOverflow=on
  Math Function : Math  Operator=square  SaturateOnIntegerOverflow=on
  Product ab (trimf) : Product  Inputs=*/  SaturateOnIntegerOverflow=on  InputSameDT=on
  Sum : Sum  Inputs=|+-  SaturateOnIntegerOverflow=on  InputSameDT=on
  Sum1 : Sum  Inputs=-+  SaturateOnIntegerOverflow=on  InputSameDT=on
  Sum9 : Sum  Inputs=-+  SaturateOnIntegerOverflow=on  InputSameDT=on
  a : Constant  Value=a
  b : Constant  Value=b
  Out1 : Outport
  wires:
  Product ab (trimf)/1 -> Math Function/1  "(x-a)/(b-a)"
  a/1 -> Sum1/1, Sum/2
  b/1 -> Sum1/2
  x/1 -> Sum/1
  Sum/1 -> Product ab (trimf)/1  "x-a"
  Sum1/1 -> Product ab (trimf)/2  "b-a"
  Constant2/1 -> Sum9/2
  Math Function/1 -> Gain1/1
  Gain1/1 -> Sum9/1
  Sum9/1 -> Out1/1  "1-2[(x-a)/(b-a)]^2"
